simulink library "csc_ldr_flir_lidar_lib"  (R2015b)
settings: Solver=ode45  SolverMode=SingleTasking  StartTime=0.0  StopTime=10.0  RelTol=1e-3
undefined symbols (not defined in the file or in its folder): pwr_ldr_on_state
libraries: simulink x2, util_common_lib x2, csc_lpr_lidar_short_long_range_pair_lib x2, util_info_lib x1
settings Model: Creator=eleanor  LastModifiedBy=Mark Agbayani
settings DataIOCC: SaveFormat=Array  SignalLoggingSaveFormat=ModelDataLogs
settings OptimizationCC: BlockReduction=off  BooleanDataType=off  ExpressionDepthLimit=2147483647
settings DebuggingCC: SaveWithParameterizedLinksMsg=none  UnderspecifiedInitializationDetection=Classic  MergeDetectMultiDrivingBlocksExec=none  SignalResolutionControl=TryResolveAllWithWarning  FcnCallInpInsideContextMsg=EnableAllAsWarning  StateNameClashWarn=warning  StrictBusMsg=Warning
settings HardwareCC: ProdBitPerPointer=32  ProdLargestAtomicFloat=None  ProdIntDivRoundTo=Undefined  ProdEndianess=Unspecified  ProdWordSize=32  ProdHWDeviceType=32-bit Generic  TargetUnknown=on
settings GRTTargetCC: GeneratePreprocessorConditionals=Disable all  CombineOutputUpdateFcns=off  GRTInterface=on
settings ConfigComp: CovModelRefEnable=Off  CovSFcnEnable=off

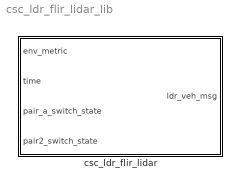
== system csc_ldr_flir_lidar_lib ==
  csc_ldr_flir_lidar : Subsystem  SystemSampleTime=0.1

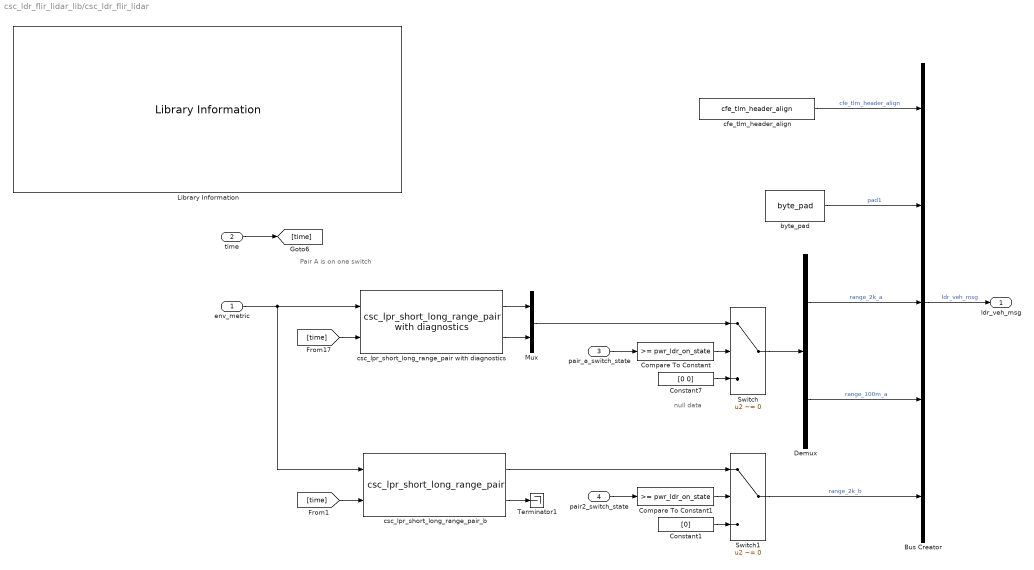
== system csc_ldr_flir_lidar_lib/csc_ldr_flir_lidar ==
  note: Pair A is on one switch
  note: null data
  env_metric : Inport
  time : Inport  Port=2
  pair_a_switch_state : Inport  Port=3
  pair2_switch_state : Inport  Port=4
  Bus Creator : BusCreator  Inputs=5  OutDataTypeStr=Bus: ldr_veh_msg  NonVirtualBus=on
  Compare To Constant : simulink/Logic and Bit Operations/Compare To Constant  relop=>=  const=pwr_ldr_on_state  OutDataTypeStr=boolean
  Compare To Constant1 : simulink/Logic and Bit Operations/Compare To Constant  relop=>=  const=pwr_ldr_on_state  OutDataTypeStr=boolean
  Constant1 : Constant  Value=[0]  OutDataTypeStr=double
  Constant7 : Constant  Value=[0 0]  OutDataTypeStr=double
  Demux : Demux  Outputs=2
  Library Information : util_info_lib/Library Information  owner='escrane'
  Mux : Mux  Inputs=2
  Switch : Switch  Criteria=u2 ~= 0
  Switch1 : Switch  Criteria=u2 ~= 0
  Terminator1 : Terminator
  byte_pad : util_common_lib/byte_pad  n_bytes=4
  cfe_tlm_header_align : util_common_lib/cfe_tlm_header_align
  csc_lpr_short_long_range_pair with diagnostics : csc_lpr_lidar_short_long_range_pair_lib/csc_lpr_short_long_range_pair with diagnostics  position_in_lander=ldr1_lander_pos  lander_dcm=ldr1_lander_dcm
  csc_lpr_short_long_range_pair_b : csc_lpr_lidar_short_long_range_pair_lib/csc_lpr_short_long_range_pair  position_in_lander=ldr2_lander_pos  lander_dcm=ldr2_lander_dcm
  ldr_veh_msg : Outport
  wires:
  Switch1/1 -> Bus Creator/5  "range_2k_b"
  Constant1/1 -> Switch1/3
  Compare To Constant1/1 -> Switch1/2
  pair2_switch_state/1 -> Compare To Constant1/1
  Constant7/1 -> Switch/3
  pair_a_switch_state/1 -> Compare To Constant/1
  Compare To Constant/1 -> Switch/2
  Switch/1 -> Demux/1
  Mux/1 -> Switch/1
  csc_lpr_short_long_range_pair with diagnostics/2 -> Mux/2
  csc_lpr_short_long_range_pair with diagnostics/1 -> Mux/1
  csc_lpr_short_long_range_pair_b/2 -> Terminator1/1
  csc_lpr_short_long_range_pair_b/1 -> Switch1/1
  [time] -> csc_lpr_short_long_range_pair_b/2
  cfe_tlm_header_align/1 -> Bus Creator/1  "cfe_tlm_header_align"
  byte_pad/1 -> Bus Creator/2  "pad1"
  time/1 -> [time]
  [time] -> csc_lpr_short_long_range_pair with diagnostics/2
  Demux/2 -> Bus Creator/4  "range_100m_a"
  env_metric/1 -> csc_lpr_short_long_range_pair with diagnostics/1, csc_lpr_short_long_range_pair_b/1
  Demux/1 -> Bus Creator/3  "range_2k_a"
  Bus Creator/1 -> ldr_veh_msg/1  "ldr_veh_msg"
